simulink model "Power_Window_Mechanism_1"  (R2014a)
settings: Solver=ode45  StartTime=0.0  StopTime=10.0  RelTol=1e-3
values from neighbouring files (symbols this model uses):
  DC_Motor_K = 0.1    [Power_Window_Mechanism_Parameters.m]
  DC_Motor_R = 0.5    [Power_Window_Mechanism_Parameters.m]
libraries: fl_lib x18, nesl_utility x4
Description:
  | Copyright 2014 The MathWorks, Inc.
settings Model: Creator=smiller  LastModifiedBy=smiller
settings DebuggingCC: UnderspecifiedInitializationDetection=Classic  StateNameClashWarn=warning

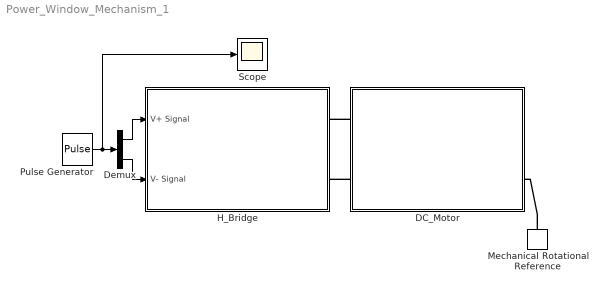
== system Power_Window_Mechanism_1 ==
  DC_Motor : Subsystem
      mask Display:
      | image(imread('Simscape_DC_Motor_IMAGE.jpg'));
      | port_label('lconn',1,'V+');
      | port_label('lconn',2,'V-');
      | port_label('rconn',1,'Shaft');
      | port_label('rconn',2,'Housing');
  Demux : Demux  Outputs=2
  H_Bridge : Subsystem
      mask Display:
      | image(imread('H_Bridge_IMAGE.jpg'));
      | port_label('Input',1,'V+ Signal');
      | port_label('Input',2,'V- Signal');
      | port_label('rconn',1,'V+');
      | port_label('rconn',2,'V-');
  Mechanical Rotational Reference : fl_lib/Mechanical/Rotational Elements/Mechanical Rotational Reference
  Pulse Generator : DiscretePulseGenerator  PulseType=Time based  Period=20  PulseWidth=50  PhaseDelay=[0 10]
  Scope : Scope
  wires:
  Pulse Generator/1 -> Scope/1, Demux/1
  Demux/1 -> H_Bridge/1(V+ Signal)
  Demux/2 -> H_Bridge/2(V- Signal)
  connections:
  DC_Motor/LConn1 -- H_Bridge/RConn1
  DC_Motor/LConn2 -- H_Bridge/RConn2
  Mechanical Rotational Reference/LConn1 -- DC_Motor/RConn2

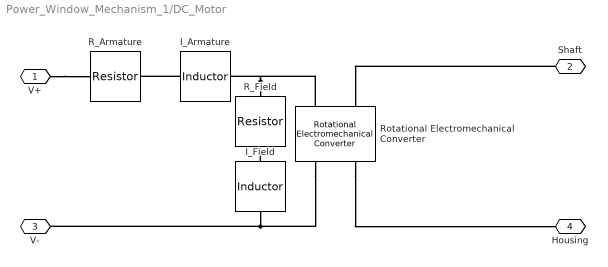
== system Power_Window_Mechanism_1/DC_Motor ==
  I_Armature : fl_lib/Electrical/Electrical Elements/Inductor  l=DC_Motor_L H  r=0 Ohm  g=1e-09 1/Ohm  i_specify=off  i_priority=High  i=0 A  v_specify=off  v_priority=High  v=0 V  i_L_specify=on  i_L_priority=High  i_L=0 A
  I_Field : fl_lib/Electrical/Electrical Elements/Inductor  l=1e-6 H  r=0 Ohm  g=1e-09 1/Ohm  i_specify=off  i_priority=High  i=0 A  v_specify=off  v_priority=High  v=0 V  i_L_specify=on  i_L_priority=High  i_L=0 A
  R_Armature : fl_lib/Electrical/Electrical Elements/Resistor  R=DC_Motor_R Ohm  i_specify=off  i_priority=High  i=0 A  v_specify=off  v_priority=High  v=0 V
  R_Field : fl_lib/Electrical/Electrical Elements/Resistor  R=1e6 Ohm  i_specify=off  i_priority=High  i=0 A  v_specify=off  v_priority=High  v=0 V
  Rotational Electromechanical Converter : fl_lib/Electrical/Electrical Elements/Rotational Electromechanical Converter  K=DC_Motor_K V/(rad/s)  i_specify=off  i_priority=High  i=0 A  v_specify=off  v_priority=High  v=0 V  t_specify=off  t_priority=High  t=0 N*m  w_specify=off  w_priority=High  w=0 rad/s
  V+ : PMIOPort  Port=1  Side=Left
  Shaft : PMIOPort  Port=2  Side=Right
  V- : PMIOPort  Port=3  Side=Left
  Housing : PMIOPort  Port=4  Side=Right
  connections:
  I_Field/LConn1 -- R_Field/RConn1
  Rotational Electromechanical Converter/RConn2 -- Housing/RConn1
  V+/RConn1 -- R_Armature/LConn1
  Shaft/RConn1 -- Rotational Electromechanical Converter/LConn2
  I_Field/RConn1 -- V-/RConn1 -- Rotational Electromechanical Converter/RConn1
  R_Field/LConn1 -- I_Armature/RConn1 -- Rotational Electromechanical Converter/LConn1
  I_Armature/LConn1 -- R_Armature/RConn1

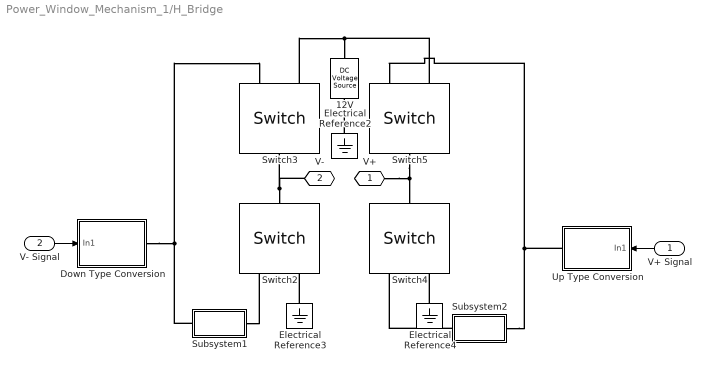
== system Power_Window_Mechanism_1/H_Bridge ==
  V+ Signal : Inport
  V- Signal : Inport  Port=2
  12V : fl_lib/Electrical/Electrical Sources/DC Voltage Source  v0=12 V
  Down Type Conversion : Subsystem
  Electrical Reference2 : fl_lib/Electrical/Electrical Elements/Electrical Reference
  Electrical Reference3 : fl_lib/Electrical/Electrical Elements/Electrical Reference
  Electrical Reference4 : fl_lib/Electrical/Electrical Elements/Electrical Reference
  Subsystem1 : Subsystem
      mask Display: disp('NOT');
  Subsystem2 : Subsystem
      mask Display: disp('NOT');
  Switch{2..5} (4 alike) : fl_lib/Electrical/Electrical Elements/Switch  R_closed=0.01 Ohm  G_open=1e-8 1/Ohm  Threshold=0  i_specify=off  i_priority=High  i=0 A  v_specify=off  v_priority=High  v=0 V
  Up Type Conversion : Subsystem
  V+ : PMIOPort  Port=1  Side=Right
  V- : PMIOPort  Port=2  Side=Right
  wires:
  V+ Signal/1 -> Up Type Conversion/1(In1)
  V- Signal/1 -> Down Type Conversion/1(In1)
  connections:
  Up Type Conversion/RConn1 -- Switch5/RConn1 -- Subsystem2/LConn1
  Subsystem2/RConn1 -- Switch4/RConn1
  Electrical Reference4/LConn1 -- Switch4/RConn2
  Subsystem1/RConn1 -- Switch2/RConn1
  Electrical Reference3/LConn1 -- Switch2/RConn2
  Electrical Reference2/LConn1 -- 12V/RConn1
  Switch2/LConn1 -- Switch3/LConn1 -- V-/RConn1
  Down Type Conversion/RConn1 -- Switch3/RConn1 -- Subsystem1/LConn1
  Switch5/RConn2 -- 12V/LConn1 -- Switch3/RConn2
  Switch5/LConn1 -- Switch4/LConn1 -- V+/RConn1

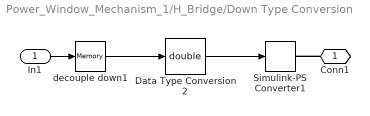
== system Power_Window_Mechanism_1/H_Bridge/Down Type Conversion ==
  In1 : Inport
  Data Type Conversion2 : DataTypeConversion  OutDataTypeStr=double
  Simulink-PS Converter1 : nesl_utility/Simulink-PS Converter  PhysicalDomain=network_engine_domain  SubClassName=ps_input  LeftPortType=input  RightPortType=output  PseudoPeriodic=off  Frequencies=[]  NoiseDistribution=none  NoiseParameters=[]  Unit=1  AffineConversion=off  InputFiltering=off  SimscapeFilterOrder=1  InputFilterTimeConstant=.001  UdotUserProvided=0
  decouple down1 : Memory
  Conn1 : PMIOPort  Port=1  Side=Right
  wires:
  Data Type Conversion2/1 -> Simulink-PS Converter1/1
  decouple down1/1 -> Data Type Conversion2/1
  In1/1 -> decouple down1/1
  connections:
  Conn1/RConn1 -- Simulink-PS Converter1/RConn1

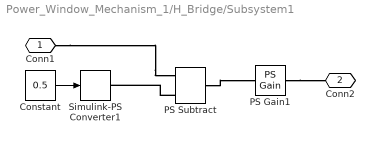
== system Power_Window_Mechanism_1/H_Bridge/Subsystem1 ==
  Constant : Constant  Value=0.5
  PS Gain1 : fl_lib/Physical Signals/Functions/PS Gain  gain=-1
  PS Subtract : fl_lib/Physical Signals/Functions/PS Subtract
  Simulink-PS Converter1 : nesl_utility/Simulink-PS Converter  PhysicalDomain=network_engine_domain  SubClassName=ps_input  LeftPortType=input  RightPortType=output  PseudoPeriodic=off  Frequencies=[]  NoiseDistribution=none  NoiseParameters=[]  Unit=1  AffineConversion=off  InputFiltering=off  SimscapeFilterOrder=1  InputFilterTimeConstant=.001  UdotUserProvided=0
  Conn1 : PMIOPort  Port=1  Side=Left
  Conn2 : PMIOPort  Port=2  Side=Right
  wires:
  Constant/1 -> Simulink-PS Converter1/1
  connections:
  PS Subtract/LConn2 -- Simulink-PS Converter1/RConn1
  Conn1/RConn1 -- PS Subtract/LConn1
  PS Subtract/RConn1 -- PS Gain1/LConn1
  PS Gain1/RConn1 -- Conn2/RConn1

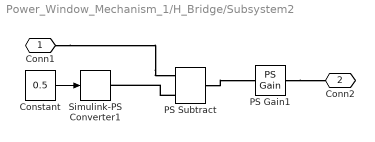
== system Power_Window_Mechanism_1/H_Bridge/Subsystem2 ==
  Constant : Constant  Value=0.5
  PS Gain1 : fl_lib/Physical Signals/Functions/PS Gain  gain=-1
  PS Subtract : fl_lib/Physical Signals/Functions/PS Subtract
  Simulink-PS Converter1 : nesl_utility/Simulink-PS Converter  PhysicalDomain=network_engine_domain  SubClassName=ps_input  LeftPortType=input  RightPortType=output  PseudoPeriodic=off  Frequencies=[]  NoiseDistribution=none  NoiseParameters=[]  Unit=1  AffineConversion=off  InputFiltering=off  SimscapeFilterOrder=1  InputFilterTimeConstant=.001  UdotUserProvided=0
  Conn1 : PMIOPort  Port=1  Side=Left
  Conn2 : PMIOPort  Port=2  Side=Right
  wires:
  Constant/1 -> Simulink-PS Converter1/1
  connections:
  PS Gain1/RConn1 -- Conn2/RConn1
  PS Subtract/RConn1 -- PS Gain1/LConn1
  Conn1/RConn1 -- PS Subtract/LConn1
  PS Subtract/LConn2 -- Simulink-PS Converter1/RConn1

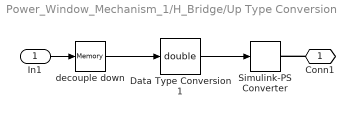
== system Power_Window_Mechanism_1/H_Bridge/Up Type Conversion ==
  In1 : Inport
  Data Type Conversion1 : DataTypeConversion  OutDataTypeStr=double
  Simulink-PS Converter : nesl_utility/Simulink-PS Converter  PhysicalDomain=network_engine_domain  SubClassName=ps_input  LeftPortType=input  RightPortType=output  PseudoPeriodic=off  Frequencies=[]  NoiseDistribution=none  NoiseParameters=[]  Unit=1  AffineConversion=off  InputFiltering=off  SimscapeFilterOrder=1  InputFilterTimeConstant=.001  UdotUserProvided=0
  decouple down : Memory
  Conn1 : PMIOPort  Port=1  Side=Right
  wires:
  Data Type Conversion1/1 -> Simulink-PS Converter/1
  decouple down/1 -> Data Type Conversion1/1
  In1/1 -> decouple down/1
  connections:
  Conn1/RConn1 -- Simulink-PS Converter/RConn1
